simulink model "Simulator_3D"  (R2018a)
settings: Solver=ode4  StartTime=0.0  StopTime=80  FixedStep=T  RelTol=1e-3
values from neighbouring files (symbols this model uses):
  A_w = 1*1.5/2    (= 0.75)    [init_Simulator.m]
  A_w2 = 1*0.27/2    (= 0.135)    [init_Simulator.m]
  epsilon_w = 0    [init_Simulator.m]
  epsilon_w2 = pi    (= 3.14159265359)    [init_Simulator.m]
  k_w = omega_w^2/g    (= 0.123862835563)    [init_Simulator.m]
  k_w2 = omega_w2^2/g    (= 0.447144836384)    [init_Simulator.m]
  Lc_0 = 7    [init_Simulator.m]
  omega_w = 2*pi/T_w    (= 1.10231321179)    [init_Simulator.m]
  omega_w2 = 2*pi/T_w2    (= 2.09439510239)    [init_Simulator.m]
  T = 1/30    (= 0.0333333333333)    [init_Simulator.m]
  w_dir = 1    [init_Simulator.m]
  w_dir2 = 1    [init_Simulator.m]
  zu_bar = X0_b(2) + Lc_0*sin(alpha_bar_0)    [init_Simulator.m]
libraries: vrlib x132
(part 6 of 6)

== system Simulator_3D/Subsystem/5 static wave points7/Subsystem12/Subsystem1 ==
  note: Aw.Sin
  t : Inport
  x : Inport  Port=2
  Constant : Constant  Value=epsilon_w2
  Gain : Gain  Gain=omega_w2
  Gain1 : Gain  Gain=k_w2
  Gain2 : Gain  Gain=A_w2
  Gain5 : Gain  Gain=A_w2*k_w2
  Sum : Sum  Inputs=++-
  Trigonometric Function : Trigonometry  Operator=sincos
  Trigonometric Function1 : Trigonometry  Operator=atan
  direction : Gain  Gain=w_dir2
  zeta(x,t) : Outport
  theta : Outport  Port=2
  wires:
  Gain/1 -> Sum/2
  Gain2/1 -> zeta(x,t)/1  "zeta(x,t)"
  Constant/1 -> Sum/1
  t/1 -> direction/1
  Gain1/1 -> Sum/3
  Trigonometric Function/1 -> Gain2/1
  x/1 -> Gain1/1
  direction/1 -> Gain/1
  Sum/1 -> Trigonometric Function/1
  Gain5/1 -> Trigonometric Function1/1
  Trigonometric Function1/1 -> theta/1
  Trigonometric Function/2 -> Gain5/1

== system Simulator_3D/Subsystem/5 static wave points7/Subsystem13/Subsystem ==
  note: Aw.Sin
  t : Inport
  x : Inport  Port=2
  Constant : Constant  Value=epsilon_w
  Gain : Gain  Gain=omega_w
  Gain1 : Gain  Gain=k_w
  Gain2 : Gain  Gain=A_w
  Gain5 : Gain  Gain=A_w*k_w
  Sum : Sum  Inputs=++-
  Trigonometric Function1 : Trigonometry  Operator=sincos
  Trigonometric Function2 : Trigonometry  Operator=atan
  direction : Gain  Gain=w_dir
  zeta(x,t) : Outport
  theta : Outport  Port=2
  wires:
  Trigonometric Function2/1 -> theta/1
  Gain5/1 -> Trigonometric Function2/1
  Trigonometric Function1/2 -> Gain5/1
  Gain/1 -> Sum/2
  Gain2/1 -> zeta(x,t)/1  "zeta(x,t)"
  Constant/1 -> Sum/1
  t/1 -> direction/1
  Gain1/1 -> Sum/3
  Trigonometric Function1/1 -> Gain2/1
  x/1 -> Gain1/1
  direction/1 -> Gain/1
  Sum/1 -> Trigonometric Function1/1

== system Simulator_3D/Subsystem/5 static wave points7/Subsystem13/Subsystem1 ==
  note: Aw.Sin
  t : Inport
  x : Inport  Port=2
  Constant : Constant  Value=epsilon_w2
  Gain : Gain  Gain=omega_w2
  Gain1 : Gain  Gain=k_w2
  Gain2 : Gain  Gain=A_w2
  Gain5 : Gain  Gain=A_w2*k_w2
  Sum : Sum  Inputs=++-
  Trigonometric Function : Trigonometry  Operator=sincos
  Trigonometric Function1 : Trigonometry  Operator=atan
  direction : Gain  Gain=w_dir2
  zeta(x,t) : Outport
  theta : Outport  Port=2
  wires:
  Trigonometric Function/2 -> Gain5/1
  Trigonometric Function1/1 -> theta/1
  Gain5/1 -> Trigonometric Function1/1
  Sum/1 -> Trigonometric Function/1
  direction/1 -> Gain/1
  x/1 -> Gain1/1
  Trigonometric Function/1 -> Gain2/1
  Gain1/1 -> Sum/3
  t/1 -> direction/1
  Constant/1 -> Sum/1
  Gain2/1 -> zeta(x,t)/1  "zeta(x,t)"
  Gain/1 -> Sum/2

== system Simulator_3D/Subsystem/5 static wave points7/Subsystem14/Subsystem ==
  note: Aw.Sin
  t : Inport
  x : Inport  Port=2
  Constant : Constant  Value=epsilon_w
  Gain : Gain  Gain=omega_w
  Gain1 : Gain  Gain=k_w
  Gain2 : Gain  Gain=A_w
  Gain5 : Gain  Gain=A_w*k_w
  Sum : Sum  Inputs=++-
  Trigonometric Function1 : Trigonometry  Operator=sincos
  Trigonometric Function2 : Trigonometry  Operator=atan
  direction : Gain  Gain=w_dir
  zeta(x,t) : Outport
  theta : Outport  Port=2
  wires:
  Sum/1 -> Trigonometric Function1/1
  direction/1 -> Gain/1
  x/1 -> Gain1/1
  Trigonometric Function1/1 -> Gain2/1
  Gain1/1 -> Sum/3
  t/1 -> direction/1
  Constant/1 -> Sum/1
  Gain2/1 -> zeta(x,t)/1  "zeta(x,t)"
  Gain/1 -> Sum/2
  Trigonometric Function1/2 -> Gain5/1
  Gain5/1 -> Trigonometric Function2/1
  Trigonometric Function2/1 -> theta/1

== system Simulator_3D/Subsystem/5 static wave points7/Subsystem14/Subsystem1 ==
  note: Aw.Sin
  t : Inport
  x : Inport  Port=2
  Constant : Constant  Value=epsilon_w2
  Gain : Gain  Gain=omega_w2
  Gain1 : Gain  Gain=k_w2
  Gain2 : Gain  Gain=A_w2
  Gain5 : Gain  Gain=A_w2*k_w2
  Sum : Sum  Inputs=++-
  Trigonometric Function : Trigonometry  Operator=sincos
  Trigonometric Function1 : Trigonometry  Operator=atan
  direction : Gain  Gain=w_dir2
  zeta(x,t) : Outport
  theta : Outport  Port=2
  wires:
  Gain/1 -> Sum/2
  Gain2/1 -> zeta(x,t)/1  "zeta(x,t)"
  Constant/1 -> Sum/1
  t/1 -> direction/1
  Gain1/1 -> Sum/3
  Trigonometric Function/1 -> Gain2/1
  x/1 -> Gain1/1
  direction/1 -> Gain/1
  Sum/1 -> Trigonometric Function/1
  Gain5/1 -> Trigonometric Function1/1
  Trigonometric Function1/1 -> theta/1
  Trigonometric Function/2 -> Gain5/1

== system Simulator_3D/Subsystem/5 static wave points7/Subsystem15/Subsystem ==
  note: Aw.Sin
  t : Inport
  x : Inport  Port=2
  Constant : Constant  Value=epsilon_w
  Gain : Gain  Gain=omega_w
  Gain1 : Gain  Gain=k_w
  Gain2 : Gain  Gain=A_w
  Gain5 : Gain  Gain=A_w*k_w
  Sum : Sum  Inputs=++-
  Trigonometric Function1 : Trigonometry  Operator=sincos
  Trigonometric Function2 : Trigonometry  Operator=atan
  direction : Gain  Gain=w_dir
  zeta(x,t) : Outport
  theta : Outport  Port=2
  wires:
  Trigonometric Function2/1 -> theta/1
  Gain5/1 -> Trigonometric Function2/1
  Trigonometric Function1/2 -> Gain5/1
  Gain/1 -> Sum/2
  Gain2/1 -> zeta(x,t)/1  "zeta(x,t)"
  Constant/1 -> Sum/1
  t/1 -> direction/1
  Gain1/1 -> Sum/3
  Trigonometric Function1/1 -> Gain2/1
  x/1 -> Gain1/1
  direction/1 -> Gain/1
  Sum/1 -> Trigonometric Function1/1

== system Simulator_3D/Subsystem/5 static wave points7/Subsystem15/Subsystem1 ==
  note: Aw.Sin
  t : Inport
  x : Inport  Port=2
  Constant : Constant  Value=epsilon_w2
  Gain : Gain  Gain=omega_w2
  Gain1 : Gain  Gain=k_w2
  Gain2 : Gain  Gain=A_w2
  Gain5 : Gain  Gain=A_w2*k_w2
  Sum : Sum  Inputs=++-
  Trigonometric Function : Trigonometry  Operator=sincos
  Trigonometric Function1 : Trigonometry  Operator=atan
  direction : Gain  Gain=w_dir2
  zeta(x,t) : Outport
  theta : Outport  Port=2
  wires:
  Trigonometric Function/2 -> Gain5/1
  Trigonometric Function1/1 -> theta/1
  Gain5/1 -> Trigonometric Function1/1
  Sum/1 -> Trigonometric Function/1
  direction/1 -> Gain/1
  x/1 -> Gain1/1
  Trigonometric Function/1 -> Gain2/1
  Gain1/1 -> Sum/3
  t/1 -> direction/1
  Constant/1 -> Sum/1
  Gain2/1 -> zeta(x,t)/1  "zeta(x,t)"
  Gain/1 -> Sum/2

== system Simulator_3D/Subsystem/5 static wave points7/Subsystem16/Subsystem ==
  note: Aw.Sin
  t : Inport
  x : Inport  Port=2
  Constant : Constant  Value=epsilon_w
  Gain : Gain  Gain=omega_w
  Gain1 : Gain  Gain=k_w
  Gain2 : Gain  Gain=A_w
  Gain5 : Gain  Gain=A_w*k_w
  Sum : Sum  Inputs=++-
  Trigonometric Function1 : Trigonometry  Operator=sincos
  Trigonometric Function2 : Trigonometry  Operator=atan
  direction : Gain  Gain=w_dir
  zeta(x,t) : Outport
  theta : Outport  Port=2
  wires:
  Sum/1 -> Trigonometric Function1/1
  direction/1 -> Gain/1
  x/1 -> Gain1/1
  Trigonometric Function1/1 -> Gain2/1
  Gain1/1 -> Sum/3
  t/1 -> direction/1
  Constant/1 -> Sum/1
  Gain2/1 -> zeta(x,t)/1  "zeta(x,t)"
  Gain/1 -> Sum/2
  Trigonometric Function1/2 -> Gain5/1
  Gain5/1 -> Trigonometric Function2/1
  Trigonometric Function2/1 -> theta/1

== system Simulator_3D/Subsystem/5 static wave points7/Subsystem16/Subsystem1 ==
  note: Aw.Sin
  t : Inport
  x : Inport  Port=2
  Constant : Constant  Value=epsilon_w2
  Gain : Gain  Gain=omega_w2
  Gain1 : Gain  Gain=k_w2
  Gain2 : Gain  Gain=A_w2
  Gain5 : Gain  Gain=A_w2*k_w2
  Sum : Sum  Inputs=++-
  Trigonometric Function : Trigonometry  Operator=sincos
  Trigonometric Function1 : Trigonometry  Operator=atan
  direction : Gain  Gain=w_dir2
  zeta(x,t) : Outport
  theta : Outport  Port=2
  wires:
  Gain/1 -> Sum/2
  Gain2/1 -> zeta(x,t)/1  "zeta(x,t)"
  Constant/1 -> Sum/1
  t/1 -> direction/1
  Gain1/1 -> Sum/3
  Trigonometric Function/1 -> Gain2/1
  x/1 -> Gain1/1
  direction/1 -> Gain/1
  Sum/1 -> Trigonometric Function/1
  Gain5/1 -> Trigonometric Function1/1
  Trigonometric Function1/1 -> theta/1
  Trigonometric Function/2 -> Gain5/1

== system Simulator_3D/Subsystem/followers/Subsystem1/Subsystem ==
  note: Aw.Sin
  t : Inport
  x : Inport  Port=2
  Constant : Constant  Value=epsilon_w
  Gain : Gain  Gain=omega_w
  Gain1 : Gain  Gain=k_w
  Gain2 : Gain  Gain=A_w
  Gain5 : Gain  Gain=A_w*k_w
  Sum : Sum  Inputs=++-
  Trigonometric Function1 : Trigonometry  Operator=sincos
  Trigonometric Function2 : Trigonometry  Operator=atan
  direction : Gain  Gain=w_dir
  zeta(x,t) : Outport
  theta : Outport  Port=2
  wires:
  Trigonometric Function2/1 -> theta/1
  Gain5/1 -> Trigonometric Function2/1
  Trigonometric Function1/2 -> Gain5/1
  Gain/1 -> Sum/2
  Gain2/1 -> zeta(x,t)/1  "zeta(x,t)"
  Constant/1 -> Sum/1
  t/1 -> direction/1
  Gain1/1 -> Sum/3
  Trigonometric Function1/1 -> Gain2/1
  x/1 -> Gain1/1
  direction/1 -> Gain/1
  Sum/1 -> Trigonometric Function1/1

== system Simulator_3D/Subsystem/followers/Subsystem1/Subsystem1 ==
  note: Aw.Sin
  t : Inport
  x : Inport  Port=2
  Constant : Constant  Value=epsilon_w2
  Gain : Gain  Gain=omega_w2
  Gain1 : Gain  Gain=k_w2
  Gain2 : Gain  Gain=A_w2
  Gain5 : Gain  Gain=A_w2*k_w2
  Sum : Sum  Inputs=++-
  Trigonometric Function : Trigonometry  Operator=sincos
  Trigonometric Function1 : Trigonometry  Operator=atan
  direction : Gain  Gain=w_dir2
  zeta(x,t) : Outport
  theta : Outport  Port=2
  wires:
  Trigonometric Function/2 -> Gain5/1
  Trigonometric Function1/1 -> theta/1
  Gain5/1 -> Trigonometric Function1/1
  Sum/1 -> Trigonometric Function/1
  direction/1 -> Gain/1
  x/1 -> Gain1/1
  Trigonometric Function/1 -> Gain2/1
  Gain1/1 -> Sum/3
  t/1 -> direction/1
  Constant/1 -> Sum/1
  Gain2/1 -> zeta(x,t)/1  "zeta(x,t)"
  Gain/1 -> Sum/2

== system Simulator_3D/Subsystem/followers/Subsystem2/Subsystem ==
  note: Aw.Sin
  t : Inport
  x : Inport  Port=2
  Constant : Constant  Value=epsilon_w
  Gain : Gain  Gain=omega_w
  Gain1 : Gain  Gain=k_w
  Gain2 : Gain  Gain=A_w
  Gain5 : Gain  Gain=A_w*k_w
  Sum : Sum  Inputs=++-
  Trigonometric Function1 : Trigonometry  Operator=sincos
  Trigonometric Function2 : Trigonometry  Operator=atan
  direction : Gain  Gain=w_dir
  zeta(x,t) : Outport
  theta : Outport  Port=2
  wires:
  Sum/1 -> Trigonometric Function1/1
  direction/1 -> Gain/1
  x/1 -> Gain1/1
  Trigonometric Function1/1 -> Gain2/1
  Gain1/1 -> Sum/3
  t/1 -> direction/1
  Constant/1 -> Sum/1
  Gain2/1 -> zeta(x,t)/1  "zeta(x,t)"
  Gain/1 -> Sum/2
  Trigonometric Function1/2 -> Gain5/1
  Gain5/1 -> Trigonometric Function2/1
  Trigonometric Function2/1 -> theta/1

== system Simulator_3D/Subsystem/followers/Subsystem2/Subsystem1 ==
  note: Aw.Sin
  t : Inport
  x : Inport  Port=2
  Constant : Constant  Value=epsilon_w2
  Gain : Gain  Gain=omega_w2
  Gain1 : Gain  Gain=k_w2
  Gain2 : Gain  Gain=A_w2
  Gain5 : Gain  Gain=A_w2*k_w2
  Sum : Sum  Inputs=++-
  Trigonometric Function : Trigonometry  Operator=sincos
  Trigonometric Function1 : Trigonometry  Operator=atan
  direction : Gain  Gain=w_dir2
  zeta(x,t) : Outport
  theta : Outport  Port=2
  wires:
  Gain/1 -> Sum/2
  Gain2/1 -> zeta(x,t)/1  "zeta(x,t)"
  Constant/1 -> Sum/1
  t/1 -> direction/1
  Gain1/1 -> Sum/3
  Trigonometric Function/1 -> Gain2/1
  x/1 -> Gain1/1
  direction/1 -> Gain/1
  Sum/1 -> Trigonometric Function/1
  Gain5/1 -> Trigonometric Function1/1
  Trigonometric Function1/1 -> theta/1
  Trigonometric Function/2 -> Gain5/1

== system Simulator_3D/Subsystem/followers/Subsystem3/Subsystem ==
  note: Aw.Sin
  t : Inport
  x : Inport  Port=2
  Constant : Constant  Value=epsilon_w
  Gain : Gain  Gain=omega_w
  Gain1 : Gain  Gain=k_w
  Gain2 : Gain  Gain=A_w
  Gain5 : Gain  Gain=A_w*k_w
  Sum : Sum  Inputs=++-
  Trigonometric Function1 : Trigonometry  Operator=sincos
  Trigonometric Function2 : Trigonometry  Operator=atan
  direction : Gain  Gain=w_dir
  zeta(x,t) : Outport
  theta : Outport  Port=2
  wires:
  Sum/1 -> Trigonometric Function1/1
  direction/1 -> Gain/1
  x/1 -> Gain1/1
  Trigonometric Function1/1 -> Gain2/1
  Gain1/1 -> Sum/3
  t/1 -> direction/1
  Constant/1 -> Sum/1
  Gain2/1 -> zeta(x,t)/1  "zeta(x,t)"
  Gain/1 -> Sum/2
  Trigonometric Function1/2 -> Gain5/1
  Gain5/1 -> Trigonometric Function2/1
  Trigonometric Function2/1 -> theta/1

== system Simulator_3D/Subsystem/followers/Subsystem3/Subsystem1 ==
  note: Aw.Sin
  t : Inport
  x : Inport  Port=2
  Constant : Constant  Value=epsilon_w2
  Gain : Gain  Gain=omega_w2
  Gain1 : Gain  Gain=k_w2
  Gain2 : Gain  Gain=A_w2
  Gain5 : Gain  Gain=A_w2*k_w2
  Sum : Sum  Inputs=++-
  Trigonometric Function : Trigonometry  Operator=sincos
  Trigonometric Function1 : Trigonometry  Operator=atan
  direction : Gain  Gain=w_dir2
  zeta(x,t) : Outport
  theta : Outport  Port=2
  wires:
  Gain/1 -> Sum/2
  Gain2/1 -> zeta(x,t)/1  "zeta(x,t)"
  Constant/1 -> Sum/1
  t/1 -> direction/1
  Gain1/1 -> Sum/3
  Trigonometric Function/1 -> Gain2/1
  x/1 -> Gain1/1
  direction/1 -> Gain/1
  Sum/1 -> Trigonometric Function/1
  Gain5/1 -> Trigonometric Function1/1
  Trigonometric Function1/1 -> theta/1
  Trigonometric Function/2 -> Gain5/1

== system Simulator_3D/Subsystem/followers/Subsystem4/Subsystem ==
  note: Aw.Sin
  t : Inport
  x : Inport  Port=2
  Constant : Constant  Value=epsilon_w
  Gain : Gain  Gain=omega_w
  Gain1 : Gain  Gain=k_w
  Gain2 : Gain  Gain=A_w
  Gain5 : Gain  Gain=A_w*k_w
  Sum : Sum  Inputs=++-
  Trigonometric Function1 : Trigonometry  Operator=sincos
  Trigonometric Function2 : Trigonometry  Operator=atan
  direction : Gain  Gain=w_dir
  zeta(x,t) : Outport
  theta : Outport  Port=2
  wires:
  Trigonometric Function2/1 -> theta/1
  Gain5/1 -> Trigonometric Function2/1
  Trigonometric Function1/2 -> Gain5/1
  Gain/1 -> Sum/2
  Gain2/1 -> zeta(x,t)/1  "zeta(x,t)"
  Constant/1 -> Sum/1
  t/1 -> direction/1
  Gain1/1 -> Sum/3
  Trigonometric Function1/1 -> Gain2/1
  x/1 -> Gain1/1
  direction/1 -> Gain/1
  Sum/1 -> Trigonometric Function1/1

== system Simulator_3D/Subsystem/followers/Subsystem4/Subsystem1 ==
  note: Aw.Sin
  t : Inport
  x : Inport  Port=2
  Constant : Constant  Value=epsilon_w2
  Gain : Gain  Gain=omega_w2
  Gain1 : Gain  Gain=k_w2
  Gain2 : Gain  Gain=A_w2
  Gain5 : Gain  Gain=A_w2*k_w2
  Sum : Sum  Inputs=++-
  Trigonometric Function : Trigonometry  Operator=sincos
  Trigonometric Function1 : Trigonometry  Operator=atan
  direction : Gain  Gain=w_dir2
  zeta(x,t) : Outport
  theta : Outport  Port=2
  wires:
  Trigonometric Function/2 -> Gain5/1
  Trigonometric Function1/1 -> theta/1
  Gain5/1 -> Trigonometric Function1/1
  Sum/1 -> Trigonometric Function/1
  direction/1 -> Gain/1
  x/1 -> Gain1/1
  Trigonometric Function/1 -> Gain2/1
  Gain1/1 -> Sum/3
  t/1 -> direction/1
  Constant/1 -> Sum/1
  Gain2/1 -> zeta(x,t)/1  "zeta(x,t)"
  Gain/1 -> Sum/2

== system Simulator_3D/Subsystem/followers/Subsystem5/Subsystem ==
  note: Aw.Sin
  t : Inport
  x : Inport  Port=2
  Constant : Constant  Value=epsilon_w
  Gain : Gain  Gain=omega_w
  Gain1 : Gain  Gain=k_w
  Gain2 : Gain  Gain=A_w
  Gain5 : Gain  Gain=A_w*k_w
  Sum : Sum  Inputs=++-
  Trigonometric Function1 : Trigonometry  Operator=sincos
  Trigonometric Function2 : Trigonometry  Operator=atan
  direction : Gain  Gain=w_dir
  zeta(x,t) : Outport
  theta : Outport  Port=2
  wires:
  Sum/1 -> Trigonometric Function1/1
  direction/1 -> Gain/1
  x/1 -> Gain1/1
  Trigonometric Function1/1 -> Gain2/1
  Gain1/1 -> Sum/3
  t/1 -> direction/1
  Constant/1 -> Sum/1
  Gain2/1 -> zeta(x,t)/1  "zeta(x,t)"
  Gain/1 -> Sum/2
  Trigonometric Function1/2 -> Gain5/1
  Gain5/1 -> Trigonometric Function2/1
  Trigonometric Function2/1 -> theta/1

== system Simulator_3D/Subsystem/followers/Subsystem5/Subsystem1 ==
  note: Aw.Sin
  t : Inport
  x : Inport  Port=2
  Constant : Constant  Value=epsilon_w2
  Gain : Gain  Gain=omega_w2
  Gain1 : Gain  Gain=k_w2
  Gain2 : Gain  Gain=A_w2
  Gain5 : Gain  Gain=A_w2*k_w2
  Sum : Sum  Inputs=++-
  Trigonometric Function : Trigonometry  Operator=sincos
  Trigonometric Function1 : Trigonometry  Operator=atan
  direction : Gain  Gain=w_dir2
  zeta(x,t) : Outport
  theta : Outport  Port=2
  wires:
  Gain/1 -> Sum/2
  Gain2/1 -> zeta(x,t)/1  "zeta(x,t)"
  Constant/1 -> Sum/1
  t/1 -> direction/1
  Gain1/1 -> Sum/3
  Trigonometric Function/1 -> Gain2/1
  x/1 -> Gain1/1
  direction/1 -> Gain/1
  Sum/1 -> Trigonometric Function/1
  Gain5/1 -> Trigonometric Function1/1
  Trigonometric Function1/1 -> theta/1
  Trigonometric Function/2 -> Gain5/1

== system Simulator_3D/Subsystem/followers/Subsystem6/Subsystem ==
  note: Aw.Sin
  t : Inport
  x : Inport  Port=2
  Constant : Constant  Value=epsilon_w
  Gain : Gain  Gain=omega_w
  Gain1 : Gain  Gain=k_w
  Gain2 : Gain  Gain=A_w
  Gain5 : Gain  Gain=A_w*k_w
  Sum : Sum  Inputs=++-
  Trigonometric Function1 : Trigonometry  Operator=sincos
  Trigonometric Function2 : Trigonometry  Operator=atan
  direction : Gain  Gain=w_dir
  zeta(x,t) : Outport
  theta : Outport  Port=2
  wires:
  Trigonometric Function2/1 -> theta/1
  Gain5/1 -> Trigonometric Function2/1
  Trigonometric Function1/2 -> Gain5/1
  Gain/1 -> Sum/2
  Gain2/1 -> zeta(x,t)/1  "zeta(x,t)"
  Constant/1 -> Sum/1
  t/1 -> direction/1
  Gain1/1 -> Sum/3
  Trigonometric Function1/1 -> Gain2/1
  x/1 -> Gain1/1
  direction/1 -> Gain/1
  Sum/1 -> Trigonometric Function1/1

== system Simulator_3D/Subsystem/followers/Subsystem6/Subsystem1 ==
  note: Aw.Sin
  t : Inport
  x : Inport  Port=2
  Constant : Constant  Value=epsilon_w2
  Gain : Gain  Gain=omega_w2
  Gain1 : Gain  Gain=k_w2
  Gain2 : Gain  Gain=A_w2
  Gain5 : Gain  Gain=A_w2*k_w2
  Sum : Sum  Inputs=++-
  Trigonometric Function : Trigonometry  Operator=sincos
  Trigonometric Function1 : Trigonometry  Operator=atan
  direction : Gain  Gain=w_dir2
  zeta(x,t) : Outport
  theta : Outport  Port=2
  wires:
  Trigonometric Function/2 -> Gain5/1
  Trigonometric Function1/1 -> theta/1
  Gain5/1 -> Trigonometric Function1/1
  Sum/1 -> Trigonometric Function/1
  direction/1 -> Gain/1
  x/1 -> Gain1/1
  Trigonometric Function/1 -> Gain2/1
  Gain1/1 -> Sum/3
  t/1 -> direction/1
  Constant/1 -> Sum/1
  Gain2/1 -> zeta(x,t)/1  "zeta(x,t)"
  Gain/1 -> Sum/2

== system Simulator_3D/Subsystem/followers/Subsystem7/Subsystem ==
  note: Aw.Sin
  t : Inport
  x : Inport  Port=2
  Constant : Constant  Value=epsilon_w
  Gain : Gain  Gain=omega_w
  Gain1 : Gain  Gain=k_w
  Gain2 : Gain  Gain=A_w
  Gain5 : Gain  Gain=A_w*k_w
  Sum : Sum  Inputs=++-
  Trigonometric Function1 : Trigonometry  Operator=sincos
  Trigonometric Function2 : Trigonometry  Operator=atan
  direction : Gain  Gain=w_dir
  zeta(x,t) : Outport
  theta : Outport  Port=2
  wires:
  Sum/1 -> Trigonometric Function1/1
  direction/1 -> Gain/1
  x/1 -> Gain1/1
  Trigonometric Function1/1 -> Gain2/1
  Gain1/1 -> Sum/3
  t/1 -> direction/1
  Constant/1 -> Sum/1
  Gain2/1 -> zeta(x,t)/1  "zeta(x,t)"
  Gain/1 -> Sum/2
  Trigonometric Function1/2 -> Gain5/1
  Gain5/1 -> Trigonometric Function2/1
  Trigonometric Function2/1 -> theta/1

== system Simulator_3D/Subsystem/followers/Subsystem7/Subsystem1 ==
  note: Aw.Sin
  t : Inport
  x : Inport  Port=2
  Constant : Constant  Value=epsilon_w2
  Gain : Gain  Gain=omega_w2
  Gain1 : Gain  Gain=k_w2
  Gain2 : Gain  Gain=A_w2
  Gain5 : Gain  Gain=A_w2*k_w2
  Sum : Sum  Inputs=++-
  Trigonometric Function : Trigonometry  Operator=sincos
  Trigonometric Function1 : Trigonometry  Operator=atan
  direction : Gain  Gain=w_dir2
  zeta(x,t) : Outport
  theta : Outport  Port=2
  wires:
  Gain/1 -> Sum/2
  Gain2/1 -> zeta(x,t)/1  "zeta(x,t)"
  Constant/1 -> Sum/1
  t/1 -> direction/1
  Gain1/1 -> Sum/3
  Trigonometric Function/1 -> Gain2/1
  x/1 -> Gain1/1
  direction/1 -> Gain/1
  Sum/1 -> Trigonometric Function/1
  Gain5/1 -> Trigonometric Function1/1
  Trigonometric Function1/1 -> theta/1
  Trigonometric Function/2 -> Gain5/1

== system Simulator_3D/Subsystem/followers/Subsystem8/Subsystem ==
  note: Aw.Sin
  t : Inport
  x : Inport  Port=2
  Constant : Constant  Value=epsilon_w
  Gain : Gain  Gain=omega_w
  Gain1 : Gain  Gain=k_w
  Gain2 : Gain  Gain=A_w
  Gain5 : Gain  Gain=A_w*k_w
  Sum : Sum  Inputs=++-
  Trigonometric Function1 : Trigonometry  Operator=sincos
  Trigonometric Function2 : Trigonometry  Operator=atan
  direction : Gain  Gain=w_dir
  zeta(x,t) : Outport
  theta : Outport  Port=2
  wires:
  Trigonometric Function2/1 -> theta/1
  Gain5/1 -> Trigonometric Function2/1
  Trigonometric Function1/2 -> Gain5/1
  Gain/1 -> Sum/2
  Gain2/1 -> zeta(x,t)/1  "zeta(x,t)"
  Constant/1 -> Sum/1
  t/1 -> direction/1
  Gain1/1 -> Sum/3
  Trigonometric Function1/1 -> Gain2/1
  x/1 -> Gain1/1
  direction/1 -> Gain/1
  Sum/1 -> Trigonometric Function1/1

== system Simulator_3D/Subsystem/followers/Subsystem8/Subsystem1 ==
  note: Aw.Sin
  t : Inport
  x : Inport  Port=2
  Constant : Constant  Value=epsilon_w2
  Gain : Gain  Gain=omega_w2
  Gain1 : Gain  Gain=k_w2
  Gain2 : Gain  Gain=A_w2
  Gain5 : Gain  Gain=A_w2*k_w2
  Sum : Sum  Inputs=++-
  Trigonometric Function : Trigonometry  Operator=sincos
  Trigonometric Function1 : Trigonometry  Operator=atan
  direction : Gain  Gain=w_dir2
  zeta(x,t) : Outport
  theta : Outport  Port=2
  wires:
  Trigonometric Function/2 -> Gain5/1
  Trigonometric Function1/1 -> theta/1
  Gain5/1 -> Trigonometric Function1/1
  Sum/1 -> Trigonometric Function/1
  direction/1 -> Gain/1
  x/1 -> Gain1/1
  Trigonometric Function/1 -> Gain2/1
  Gain1/1 -> Sum/3
  t/1 -> direction/1
  Constant/1 -> Sum/1
  Gain2/1 -> zeta(x,t)/1  "zeta(x,t)"
  Gain/1 -> Sum/2
